simulink model "simscape_full"  (R2024b)
settings: Solver=ode23t  StartTime=0.0  StopTime=stopTime  FixedStep=timestep  MaxStep=2
values from neighbouring files (symbols this model uses):
  timestep = 0.5    [design_details.m]
libraries: aircraft_refuel_control x1, simulink x1, GS_refuel_control x1
settings Model: Creator=MW  LastModifiedBy=MW
settings SolverCC: MaxConsecutiveMinStep=6  DaesscMode=Robust  SolverResetMethod=Robust
settings ModelReferenceCC: UpdateModelReferenceTargets=IfOutOfDate
settings SFSimCC: SFSimEcho=off  SimTargetLang=C++
settings SimscapeCC: SimscapeLogType=all  SimscapeLogSimulationStatistics=on  SimscapeLogLimitData=off

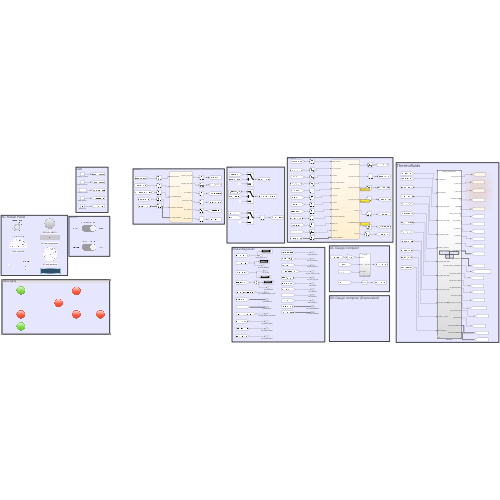
[thumbnail: Simulink's stored preview of the top-level diagram]
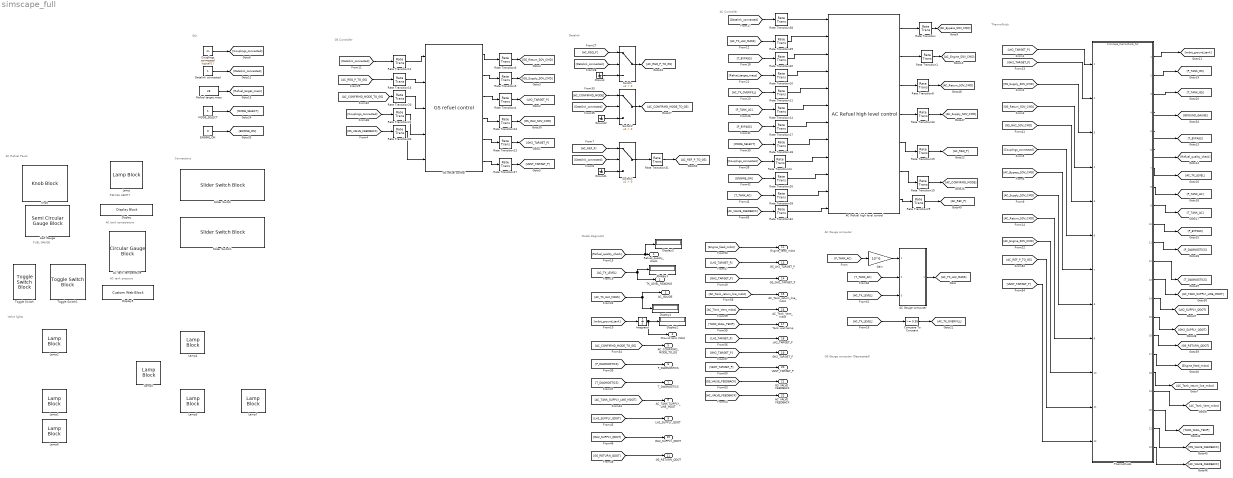
== system simscape_full ==
  note: Valve lights
  note: REFUEL ABORT
  note: AC tank pressure
  note: AC Refuel Panel
  note: GUI
  note: Connections
  note: AC tank temperature
  note: FUEL GAUGE
  note: Model diagnostic
  note: GS Gauge computer (Deprecated)
  note: Datalink
  note: Thermofluids
  note: AC Controller
  note: AC Gauge computer
  note: GS Controller
  AC Gauge computer : Subsystem  ReferencedSubsystem=AC_gauge
  AC Refuel high level control : aircraft_refuel_control/AC Refuel high level control  SystemSampleTime=timestep  VariantActivationTime=update diagram  AllowFlexibleInterface=on  Latency=0  AutoFrameSizeCalculation=off
  AC tank temperature : CircularGaugeBlock  LabelPosition=Hide  ScaleMax=0.7
  Compare To Constant : simulink/Logic and Bit Operations/Compare To Constant  relop=>=  const=0.95  OutDataTypeStr=boolean
  Couplings connected : Constant  Value=logical(1)
  Datalink connected : Constant
  Display : DisplayBlock  LabelPosition=Hide  Transparency=1
  Display{1..4} (4 alike) : Display
  Display5 : CustomWebBlock  LabelPosition=Hide  ShowInitialText=on  Configuration="{\"components\":[{\"name\":\"DisplayComponent\",\"settings\":{\"bold\":false,\"font\":\"DSEG7 Classic\",\"fontColor\":[255,255,200],\"fontSize\":\"14\",\"format\":\"short\",\"formatString\":\"%d\",\"italic\":false,\"position\":[0,0,1,1],\"underline\":false}},{\"name\":\"BackgroundImageComponent\",\"settings\":{\"image\":{\"size\":[300,80],\"src\":\"data:image\\/svg+xml;base64,PHN2ZyBpZD0iZnJhbWUiIHhtbG5zPSJodHRwOi8vd3d3LnczLm9yZy8yMDAwL3N2ZyIgeG1sbnM6eGxpbms9Imh0dHA6Ly93d3cudzMub3JnLzE5OTkveGxpbmsiIHZpZXdCb3g9IjAgMCAzODAgMTAxIj48ZGVmcz48c3R5bGU+LmNscy0xe2ZpbGw6IzAwMmI0Mjt9LmNscy0ye2ZpbGw6IzQyNzA4Mjt9LmNscy0ze2ZpbGw6dXJsKCNyYWRpYWwtZ3JhZGllbnQpO308L3N0eWxlPjxyYWRpYWxHcmFkaWVudCBpZD0icmFkaWFsLWdyYWRpZW50IiBjeD0iMTkwIiBjeT0iNTAuNSIgcj0iMjY5LjIxIiBncmFkaWVudFVuaXRzPSJ1c2VyU3BhY2VPblVzZSI+PHN0b3Agb2Zmc2V0PSIwLjAxIiBzdG9wLWNvbG9yPSIjM2U0ZjU4Ii8+PHN0b3Agb2Zmc2V0PSIwLjA2IiBzdG9wLWNvbG9yPSIjNDQ1NzYxIi8+PHN0b3Agb2Zmc2V0PSIwLjE1IiBzdG9wLWNvbG9yPSIjNTU2YTc2Ii8+PHN0b3Agb2Zmc2V0PSIwLjI1IiBzdG9wLWNvbG9yPSIjNmQ4ODk1Ii8+PHN0b3Agb2Zmc2V0PSIwLjM4IiBzdG9wLWNvbG9yPSIjOGZiMmMzIi8+PHN0b3Agb2Zmc2V0PSIwLjUyIiBzdG9wLWNvbG9yPSIjYjZlNGZhIi8+PHN0b3Agb2Zmc2V0PSIxIiBzdG9wLWNvbG9yPSIjMTU0NjU3Ii8+PC9yYWRpYWxHcmFkaWVudD48L2RlZnM+PGcgaWQ9IkxheWVyXzIiIGRhdGEtbmFtZT0iTGF5ZXIgMiI+PGcgaWQ9IkxheWVyXzEtMiIgZGF0YS1uYW1lPSJMYXllciAxLTIiPjxyZWN0IGlkPSJyZWN0MTAzNiIgY2xhc3M9ImNscy0xIiB4PSIxMSIgeT0iMTEiIHdpZHRoPSIzNTgiIGhlaWdodD0iNzkiLz48cGF0aCBpZD0icGF0aDEwMzgiIGNsYXNzPSJjbHMtMiIgZD0iTTgsOFY5M0gzNzJWOFpNMzY5LDkwSDExVjExSDM2OVoiLz48cGF0aCBpZD0icGF0aDEwNDAiIGNsYXNzPSJjbHMtMyIgZD0iTTAsMFYxMDFIMzgwVjBaTTM3Miw5M0g4VjhIMzcyWiIvPjwvZz48L2c+PC9zdmc+\",\"srcOrientation\":\"Right\"},\"position\":[0,0,1,1],\"scaleMode\":\"0\"}},{\"name\":\"ForegroundImageComponent\",\"settings\":{\"angle\":0,\"image\":{\"size\":[0,0],\"src\":\"default\"},\"isForeground\":1,\"position\":[0,0,1,1],\"scaleMode\":\"0\"}}],\"settings\":{\"BindingType\":\"signal\",\"aspectRatio\":1.032258064516129,\"backgroundColor\":[0,0,0,\"1\"],\"backgroundOffset\":0.14,\"backgroundOpacity\":1,\"fixedAspectRatio\":\"on\",\"showBackgroundColor\":false,\"value\":0,\"version\":\"R2023b\"},\"type\":\"Display\"}"
  ENGINE_ON : Constant  Value=0
  GS refuel control : GS_refuel_control/GS refuel control  SystemSampleTime=timestep  VariantActivationTime=update diagram  AllowFlexibleInterface=on  Latency=0  AutoFrameSizeCalculation=off
  Gain : Gain  Gain=10^6
  Ground : Ground
  Ground1 : Ground
  Ground2 : Ground
  Half Gauge : SemiCircularGaugeBlock  ScaleMax=35
  Integrator : Integrator
  Knob : KnobBlock  ScaleMax=28
  Lamp{,1..7} (8 alike) : LampBlock  LabelPosition=Hide
  MODE_SELECT : Constant
  Rate Transition{,1,4..6,8,10..21,23..24,26..33,38..40} (31 alike) : RateTransition
  Refuel target mass : Constant  Value=28
  Slider Switch : SliderSwitchBlock
      settings: Values={{'Disconnected', 'Connected'}, [0 1]}
  Slider Switch1 : SliderSwitchBlock
      settings: Values={{'Disconnected', 'Connected'}, [0 1]}
  Switch : Switch  Criteria=u2 > Threshold  SaturateOnIntegerOverflow=off  InputSameDT=off
  Switch1 : Switch  Criteria=u2 > Threshold  OutDataTypeStr=double  SaturateOnIntegerOverflow=off  InputSameDT=off
  Switch2 : Switch  Criteria=u2 > Threshold  SaturateOnIntegerOverflow=off  InputSameDT=off
  Thermofluids : ModelReference  ModelNameDialog=simscape_thermofluids_full.slx  SimulationMode=Normal  ModelReferenceVersion=1.461
  Toggle Switch : ToggleSwitchBlock
      settings: Values={{'DEFUEL', 'REFUEL'}, [0 1]}
  Toggle Switch1 : ToggleSwitchBlock
      settings: Values={{'ENGINE_SHUTDOWN', 'ENGINE_START'}, [0 1]}
  Refuel_quality_check : Outport
  TK_LEVEL_READING : Outport  Port=2
  AC_GAUGE : Outport  Port=3
  Ground tank Mdot : Outport  Port=4
  AC_CONFIRMD_MODE_TO_GS : Outport  Port=5
  P_DIAGNOSTICS : Outport  Port=6  OutDataTypeStr=Bus: P_DIAGNOSTIC
  T_DIAGNOSTICS : Outport  Port=7  OutDataTypeStr=Bus: T_DIAGNOSTIC
  AC_TANK_SUPPLY_LINE_MDOT : Outport  Port=8
  LH2_SUPPLY_QDOT : Outport  Port=9
  GH2_SUPPLY_QDOT : Outport  Port=10
  GS_RETURN_QDOT : Outport  Port=11
  Engine_feed_mdot : Outport  Port=12
  GS_LH2_TARGET_P : Outport  Port=13
  GS_GH2_TARGET_P : Outport  Port=14
  AC_Tank_return_line_mdot : Outport  Port=15
  AC_Tank_Vent_mdot : Outport  Port=16
  Tank wall temp : Outport  Port=17
  LH2_TARGET_P : Outport  Port=18
  GH2_TARGET_P : Outport  Port=19
  VENT_TARGET_P : Outport  Port=20
  GS_VALVE_FEEDBACK : Outport  Port=21  OutDataTypeStr=Bus: GS_VALVE_FEEDBACK
  AC_VALVE_FEEDBACK : Outport  Port=22  OutDataTypeStr=Bus: AC_VALVE_FEEDBACK
  wires:
  Couplings connected/1 -> [Couplings_connected]
  Datalink connected/1 -> [Datalink_connected]
  Refuel target mass/1 -> [Refuel_target_mass]
  MODE_SELECT/1 -> [MODE_SELECT]
  ENGINE_ON/1 -> [ENGINE_ON]
  Thermofluids/21 -> [GS_VALVE_FEEDBACK]
  Thermofluids/22 -> [AC_VALVE_FEEDBACK]
  [AC_VALVE_FEEDBACK] -> Rate Transition32/1
  [GS_VALVE_FEEDBACK] -> GS_VALVE_FEEDBACK/1
  [AC_VALVE_FEEDBACK] -> AC_VALVE_FEEDBACK/1
  Switch/1 -> [AC_REQ_P_TO_GS]
  [P_DIAGNOSTICS] -> P_DIAGNOSTICS/1
  Thermofluids/11 -> [P_DIAGNOSTICS]
  Thermofluids/15 -> [GH2_SUPPLY_QDOT]
  [P_TANK_AC] -> Rate Transition14/1
  Rate Transition33/1 -> [AC_Supply_SOV_CMD]
  [Refuel_quality_check] -> Display3/1, Refuel_quality_check/1
  Rate Transition39/1 -> AC Refuel high level control/2
  Thermofluids/10 -> [P_BYPASS]
  [AC_REF_P_TO_GS] -> Thermofluids/11
  [AC_REQ_P] -> Switch/1
  [Engine_feed_mdot] -> Engine_feed_mdot/1
  Thermofluids/4 -> [GROUND_GAUGE]
  [GS_Supply_SOV_CMD] -> Thermofluids/3
  AC Refuel high level control/7 -> Rate Transition29/1
  Rate Transition17/1 -> AC Refuel high level control/7
  Integrator/1 -> Ground tank Mdot/1, Display2/1
  Rate Transition14/1 -> AC Refuel high level control/6
  [GH2_SUPPLY_QDOT] -> GH2_SUPPLY_QDOT/1
  Thermofluids/3 -> [T_TANK_GS]
  [AC_Engine_SOV_CMD] -> Thermofluids/10
  Rate Transition26/1 -> AC Refuel high level control/10
  Thermofluids/9 -> [T_TANK_AC]
  AC Refuel high level control/1 -> Rate Transition/1
  Ground/1 -> Switch/3
  [GH2_TARGET_P] -> GS_GH2_TARGET_P/1
  AC Gauge computer/1 -> [AC_TK_LH2_MASS]
  Thermofluids/20 -> [TANK_WALL_TEMP]
  Rate Transition8/1 -> [AC_Return_SOV_CMD]
  [AC_TK_LEVEL] -> Compare To Constant/1
  [Couplings_connected] -> Rate Transition24/1
  Ground1/1 -> Switch1/3
  [GH2_TARGET_P] -> GH2_TARGET_P/1
  [P_TANK_AC] -> Gain/1
  [AC_TK_LH2_MASS] -> Rate Transition39/1
  Thermofluids/17 -> [Engine_feed_mdot]
  Thermofluids/8 -> [P_TANK_AC]
  AC Refuel high level control/2 -> Rate Transition1/1
  AC Refuel high level control/4 -> Rate Transition33/1
  [AC_Tank_Vent_mdot] -> AC_Tank_Vent_mdot/1
  [AC_Bypass_SOV_CMD] -> Thermofluids/7
  Rate Transition28/1 -> AC Refuel high level control/11
  [GS_RETURN_QDOT] -> GS_RETURN_QDOT/1
  AC Refuel high level control/5 -> Rate Transition15/1
  [T_BYPASS] -> Rate Transition40/1
  Thermofluids/16 -> [GS_RETURN_QDOT]
  [Datalink_connected] -> Rate Transition38/1
  Thermofluids/1 -> [mdot_ground_tank]
  Rate Transition15/1 -> [AC_REQ_P]
  Ground2/1 -> Switch2/3
  [VENT_TARGET_P] -> VENT_TARGET_P/1
  [AC_CONFIRMD_MODE] -> Switch2/1
  [LH2_TARGET_P] -> Thermofluids/1
  Rate Transition10/1 -> AC Refuel high level control/4
  [AC_Supply_SOV_CMD] -> Thermofluids/8
  [VENT_TARGET_P] -> Thermofluids/12
  [mdot_ground_tank] -> Integrator/1
  Thermofluids/19 -> [AC_Tank_Vent_mdot]
  [GS_Return_SOV_CMD] -> Thermofluids/4
  Rate Transition29/1 -> [AC_REF_P]
  Rate Transition18/1 -> AC Refuel high level control/8
  Thermofluids/13 -> [AC_TANK_SUPPLY_LINE_MDOT]
  Thermofluids/18 -> [AC_Tank_return_line_mdot]
  [P_BYPASS] -> Rate Transition17/1
  Compare To Constant/1 -> [AC_TK_OVERFILL]
  [LH2_SUPPLY_QDOT] -> LH2_SUPPLY_QDOT/1
  Switch1/1 -> Rate Transition31/1
  [AC_REF_P] -> Switch1/1
  Rate Transition19/1 -> [AC_CONFIRMD_MODE]
  [AC_TK_LEVEL] -> AC Gauge computer/3
  [AC_Return_SOV_CMD] -> Thermofluids/9
  [GH2_TARGET_P] -> Thermofluids/2
  Rate Transition1/1 -> [AC_Engine_SOV_CMD]
  Thermofluids/14 -> [LH2_SUPPLY_QDOT]
  [MODE_SELECT] -> Rate Transition18/1
  [GS_GH2_SOV_CMD] -> Thermofluids/5
  [T_TANK_AC] -> Rate Transition28/1
  Gain/1 -> AC Gauge computer/1
  Rate Transition24/1 -> AC Refuel high level control/9
  Rate Transition38/1 -> AC Refuel high level control/1
  [Datalink_connected] -> Switch1/2
  Thermofluids/12 -> [T_DIAGNOSTICS]
  Rate Transition31/1 -> [AC_REF_P_TO_GS]
  [AC_CONFIRMD_MODE_TO_GS] -> AC_CONFIRMD_MODE_TO_GS/1
  [AC_TANK_SUPPLY_LINE_MDOT] -> AC_TANK_SUPPLY_LINE_MDOT/1
  [AC_Tank_return_line_mdot] -> AC_Tank_return_line_mdot/1
  [ENGINE_ON] -> Rate Transition26/1
  Thermofluids/5 -> [T_BYPASS]
  [TANK_WALL_TEMP] -> Tank wall temp/1
  Switch2/1 -> [AC_CONFIRMD_MODE_TO_GS]
  [T_TANK_AC] -> AC Gauge computer/2
  Thermofluids/7 -> [AC_TK_LEVEL]
  [AC_TK_OVERFILL] -> Rate Transition11/1
  [AC_TK_LH2_MASS] -> Display4/1, AC_GAUGE/1
  [Datalink_connected] -> Switch2/2
  Rate Transition40/1 -> AC Refuel high level control/3
  Rate Transition/1 -> [AC_Bypass_SOV_CMD]
  [AC_TK_LEVEL] -> Display1/1, TK_LEVEL_READING/1
  [Refuel_target_mass] -> Rate Transition10/1
  Thermofluids/2 -> [P_TANK_GS]
  Rate Transition11/1 -> AC Refuel high level control/5
  [Couplings_connected] -> Thermofluids/6
  [LH2_TARGET_P] -> GS_LH2_TARGET_P/1
  Thermofluids/6 -> [Refuel_quality_check]
  [LH2_TARGET_P] -> LH2_TARGET_P/1
  Rate Transition32/1 -> AC Refuel high level control/12
  AC Refuel high level control/6 -> Rate Transition19/1
  [T_DIAGNOSTICS] -> T_DIAGNOSTICS/1
  AC Refuel high level control/3 -> Rate Transition8/1
  [Datalink_connected] -> Switch/2
  Rate Transition30/1 -> GS refuel control/5
  [GS_VALVE_FEEDBACK] -> Rate Transition30/1
  Rate Transition13/1 -> [GH2_TARGET_P]
  [Datalink_connected] -> Rate Transition12/1
  GS refuel control/6 -> Rate Transition27/1
  GS refuel control/1 -> Rate Transition6/1
  Rate Transition12/1 -> GS refuel control/1
  Rate Transition6/1 -> [GS_Return_SOV_CMD]
  [AC_REQ_P_TO_GS] -> Rate Transition16/1
  Rate Transition16/1 -> GS refuel control/2
  Rate Transition21/1 -> GS refuel control/4
  [AC_CONFIRMD_MODE_TO_GS] -> Rate Transition20/1
  Rate Transition5/1 -> [GS_Supply_SOV_CMD]
  GS refuel control/4 -> Rate Transition23/1
  Rate Transition23/1 -> [GS_GH2_SOV_CMD]
  Rate Transition20/1 -> GS refuel control/3
  [Couplings_connected] -> Rate Transition21/1
  GS refuel control/2 -> Rate Transition5/1
  GS refuel control/3 -> Rate Transition4/1
  GS refuel control/5 -> Rate Transition13/1
  Rate Transition27/1 -> [VENT_TARGET_P]
  Rate Transition4/1 -> [LH2_TARGET_P]
